simulink model "non_linear_2"  (R2018a)
settings: Solver=VariableStepAuto  StartTime=0.0  StopTime=16.0  RelTol=1e-3
settings Model: Creator=ASUS  LastModifiedBy=ASUS

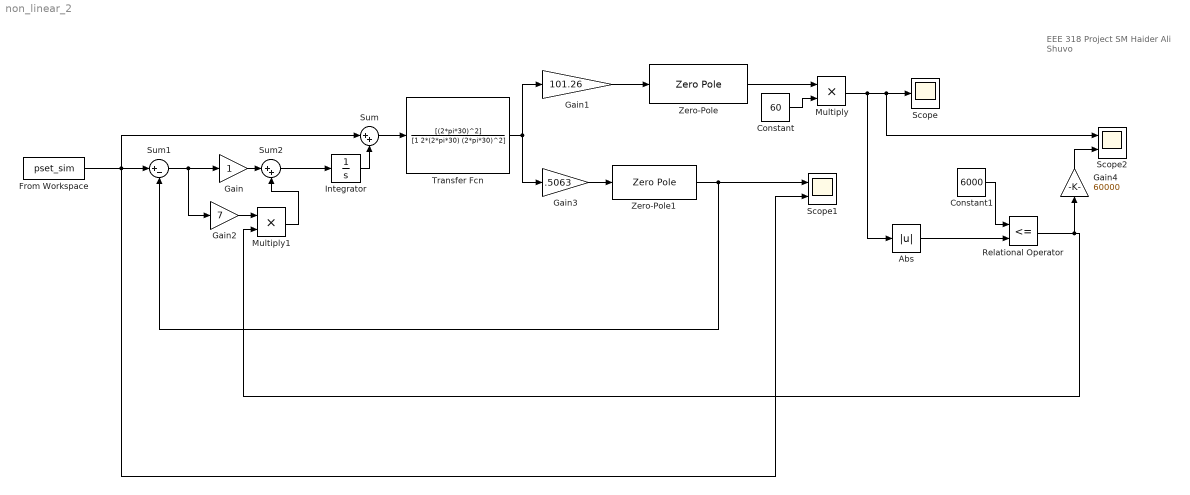
== system non_linear_2 ==
  note: EEE 318 Project
      | SM Haider Ali Shuvo
  Abs : Abs
  Constant : Constant  Value=60
  Constant1 : Constant  Value=6000
  From Workspace : FromWorkspace  VariableName=pset_sim  SampleTime=0
  Gain : Gain
  Gain1 : Gain  Gain=101.26
  Gain2 : Gain  Gain=7
  Gain3 : Gain  Gain=.5063
  Gain4 : Gain  Gain=60000
  Integrator : Integrator
  Multiply : Product
  Multiply1 : Product
  Relational Operator : RelationalOperator  Operator=<=  OutDataTypeStr=boolean  RndMeth=Simplest
  Scope : Scope
  Scope1 : Scope  NumInputPorts=2
  Scope2 : Scope  NumInputPorts=2
  Sum : Sum  Inputs=|++
  Sum1 : Sum  Inputs=|+-
  Sum2 : Sum  Inputs=|++
  Transfer Fcn : TransferFcn  Numerator=[(2*pi*30)^2]  Denominator=[1 2*(2*pi*30) (2*pi*30)^2]
  Zero-Pole : ZeroPole  Zeros=[-8.88e-16]  Poles=[-5.4436]
  Zero-Pole1 : ZeroPole  Zeros=[-10]  Poles=[-5.4436]
  wires:
  From Workspace/1 -> Scope1/2, Sum/1, Sum1/1
  Gain3/1 -> Zero-Pole1/1
  Constant/1 -> Multiply/2
  Sum1/1 -> Gain2/1, Gain/1
  Multiply/1 -> Abs/1, Scope2/1, Scope/1
  Gain1/1 -> Zero-Pole/1
  Transfer Fcn/1 -> Gain3/1, Gain1/1
  Integrator/1 -> Sum/2
  Sum/1 -> Transfer Fcn/1
  Zero-Pole1/1 -> Scope1/1, Sum1/2
  Zero-Pole/1 -> Multiply/1
  Constant1/1 -> Relational Operator/1
  Gain2/1 -> Multiply1/1
  Gain/1 -> Sum2/1
  Multiply1/1 -> Sum2/2
  Sum2/1 -> Integrator/1
  Relational Operator/1 -> Multiply1/2, Gain4/1
  Gain4/1 -> Scope2/2
  Abs/1 -> Relational Operator/2
